simulink model "Example_4_4"  (R2021b)
settings: Solver=VariableStepAuto  StartTime=0.0  StopTime=10.0  RelTol=1e-3
settings Model: Creator=saeed  LastModifiedBy=saeed

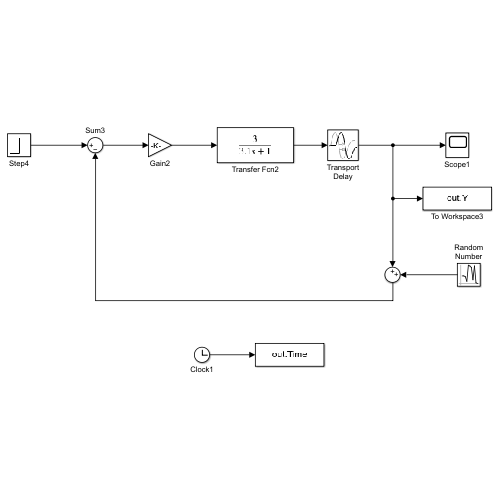
[thumbnail: Simulink's stored preview of the top-level diagram]
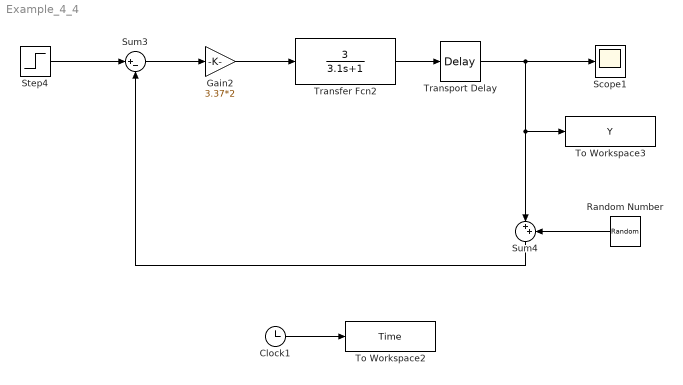
== system Example_4_4 ==
  Clock1 : Clock
  Gain2 : Gain  Gain=3.37*2
  Random Number : RandomNumber  Variance=0.15  Seed=061233  SampleTime=0
  Scope1 : Scope
  Step4 : Step  Time=0  After=30  SampleTime=0
  Sum3 : Sum  Inputs=|+-
  Sum4 : Sum  Inputs=|++
  To Workspace2 : ToWorkspace  VariableName=Time  SaveFormat=Timeseries  SampleTime=-1
  To Workspace3 : ToWorkspace  VariableName=Y  SaveFormat=Timeseries  SampleTime=-1
  Transfer Fcn2 : TransferFcn  Numerator=[3]  Denominator=[3.1 1]
  Transport Delay : TransportDelay  DelayTime=0.15
  wires:
  Clock1/1 -> To Workspace2/1
  Step4/1 -> Sum3/1
  Sum3/1 -> Gain2/1
  Sum4/1 -> Sum3/2
  Random Number/1 -> Sum4/2
  Transfer Fcn2/1 -> Transport Delay/1
  Gain2/1 -> Transfer Fcn2/1
  Transport Delay/1 -> To Workspace3/1, Sum4/1, Scope1/1
